simulink model "etNavn"  (R2021b)
settings: Solver=VariableStepAuto  StartTime=0.0  StopTime=6  RelTol=1e-3
settings Model: Creator=probo  LastModifiedBy=Elias

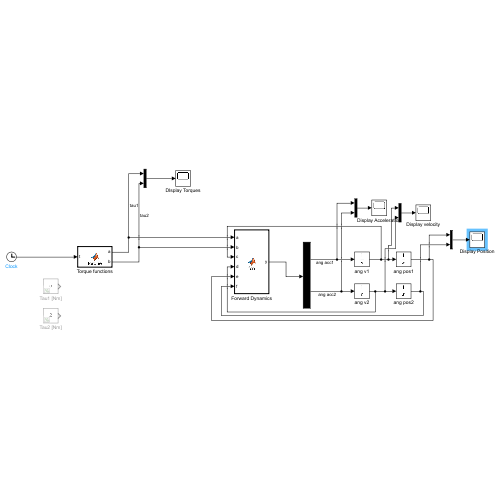
[thumbnail: Simulink's stored preview of the top-level diagram]
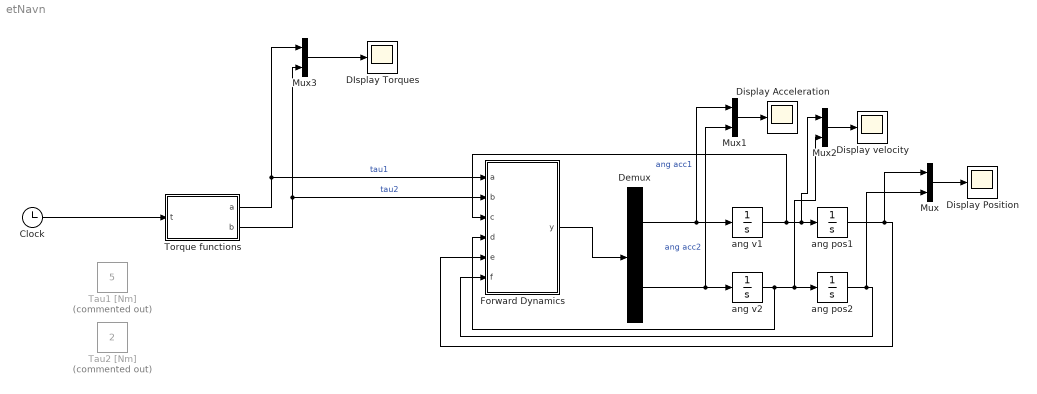
== system etNavn ==
  Clock : Clock
  DIsplay Torques : Scope
  Demux : Demux  Outputs=2
  Display Acceleration : Scope
  Display Position : Scope
  Display velocity : Scope
  Forward Dynamics : MATLAB Function  TreatAsAtomicUnit=on
  Mux{,1..3} (4 alike) : Mux  Inputs=2
  Tau1 [Nm] : Constant  Commented=on  Value=5
  Tau2 [Nm] : Constant  Commented=on  Value=2
  Torque functions : MATLAB Function  TreatAsAtomicUnit=on
  ang pos1 : Integrator
  ang pos2 : Integrator
  ang v1 : Integrator
  ang v2 : Integrator
  wires:
  Forward Dynamics/1(y) -> Demux/1
  Demux/1 -> Mux1/1, ang v1/1  "ang acc1"
  Demux/2 -> Mux1/2, ang v2/1  "ang acc2"
  ang v1/1 -> Forward Dynamics/3(c), Mux2/1, ang pos1/1
  ang v2/1 -> Forward Dynamics/4(d), ang pos2/1, Mux2/2
  ang pos2/1 -> Mux/2, Forward Dynamics/6(f)
  ang pos1/1 -> Mux/1, Forward Dynamics/5(e)
  Mux1/1 -> Display Acceleration/1
  Mux2/1 -> Display velocity/1
  Torque functions/2(b) -> Forward Dynamics/2(b), Mux3/2  "tau2"
  Torque functions/1(a) -> Forward Dynamics/1(a), Mux3/1  "tau1"
  Mux3/1 -> DIsplay Torques/1
  Clock/1 -> Torque functions/1(t)
  Mux/1 -> Display Position/1

== matlab function etNavn/Torque functions ==
  data: t input; a output; b output
function [a,b] = torque(t)

u = [0, 0];

if t <= 3
    a = 2*t
    b = (35/30)*t
else
    a = -2*t+12
    b = -(35/30)*t+7
end

== matlab function etNavn/Forward Dynamics ==
  data: a input; y output; b input; c input; d input; e input; f input
function y = fcn(a, b, c, d, e, f)

% Torques

tau1 = a;
tau2 = b;

% Joint Velocity & Position

dtheta1 = c;
theta1 = e;

dtheta2 = d;
theta2 = f;

%Variables for link 1
l1 = 0.5;
m1 = 4.6;
I1= (1/12)*m1*l1^2;
Sc1 = [(l1/2)*cos(theta1); (l1/2)*sin(theta1); 0];

Vc1 = diff(Sc1);
dVc1 = diff(Vc1);

%Variables for link 2
l2 = 0.5;
m2 = 2.3;
I2 = (1/12)*m2*l2^2;
Sc2 = [(l2/2)*cos(theta1+theta2); (l2/2)*sin(theta1+theta2); 0];
lc2 = l2/2;

Vc2 = [-l1*dtheta1*sin(theta1)-(dtheta1+dtheta2)*lc2*sin(theta1+theta2); l1*dtheta1*cos(theta1)+(dtheta1+dtheta2)*lc2*cos(theta1+theta2); 0];
dVc2 = diff(Vc2);

% Global variables

g = [0     ;
     -9.81];

S1 = [l1*cos(theta1); l1*sin(theta1)];
S2 = [l2*cos(theta1+theta2); l2*sin(theta1+theta2)];

% Functions

ddtheta1 = (1/I1)*(tau1-tau2-planarCross(Sc1, m1*Vc1) + planarCross(Sc1, m1*g) - planarCross(S1, m2*Vc2) + planarCross(S1, m2*g));

ddtheta2 = (1/I2)*(tau2 - planarCross(Sc2, (m2*Vc2 - m2*g(2)))-ddtheta1);

y = [ddtheta1;
     ddtheta2];
